simulink model "ex6simb"  (R2015a)
settings: Solver=ode45  StartTime=0.0  StopTime=10.0  RelTol=1e-3
values from neighbouring files (symbols this model uses):
  den = G.den{1}'    [s2z.m]
  num = G.num{1}'    [s2z.m]
  Ts = 0.1    [ex3.m]
undefined symbols (not defined in the file or in its folder): den_pade, num_pade
settings Model: Creator=brunopeixoto  LastModifiedBy=brunopeixoto

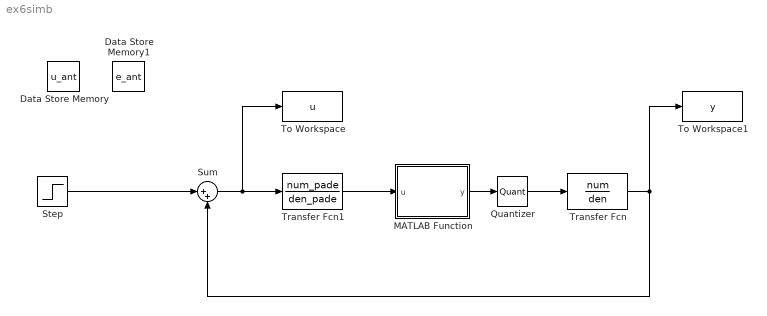
== system ex6simb ==
  Data Store Memory : DataStoreMemory  DataStoreName=u_ant  OutDataTypeStr=double
  Data Store Memory1 : DataStoreMemory  DataStoreName=e_ant  OutDataTypeStr=double
  MATLAB Function : MATLAB Function  TreatAsAtomicUnit=on  SystemSampleTime=Ts
  Quantizer : Quantizer
  Step : Step  SampleTime=0
  Sum : Sum  Inputs=|++
  To Workspace : ToWorkspace  VariableName=u  SaveFormat=Structure With Time  SampleTime=-1
  To Workspace1 : ToWorkspace  VariableName=y  SaveFormat=Structure With Time  SampleTime=-1
  Transfer Fcn : TransferFcn  Numerator=num  Denominator=den
  Transfer Fcn1 : TransferFcn  Numerator=num_pade  Denominator=den_pade
  wires:
  MATLAB Function/1(y) -> Quantizer/1
  Quantizer/1 -> Transfer Fcn/1
  Transfer Fcn/1 -> Sum/2, To Workspace1/1
  Step/1 -> Sum/1
  Sum/1 -> Transfer Fcn1/1, To Workspace/1
  Transfer Fcn1/1 -> MATLAB Function/1(u)

== matlab function ex6simb/MATLAB Function ==
  settings: updateMethod=DISCRETE  sampleTime=Ts
  data: u input; y output; param parameter; u_ant data_store_memory
function y = fcn(u, param)
%#codegen
global u_ant; global e_ant;

Cz = param(1);
Ts = Cz.ts;



y = u;
